simulink model "APCSBussedVersion"  (R2023a)
settings: Solver=VariableStepAuto  StartTime=0.0  StopTime=10.0  RelTol=1e-3
settings Model: Creator=asd19005  LastModifiedBy=asd19005

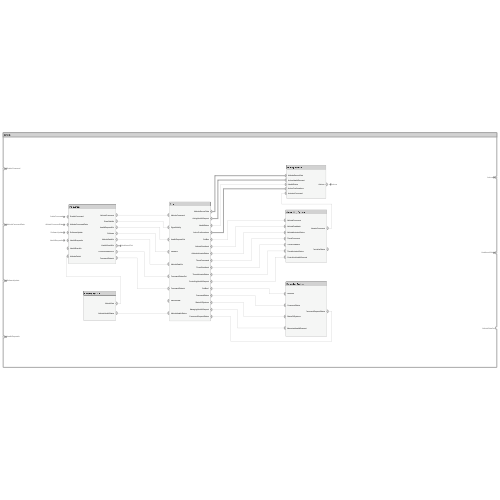
[thumbnail: Simulink's stored preview of the top-level diagram]
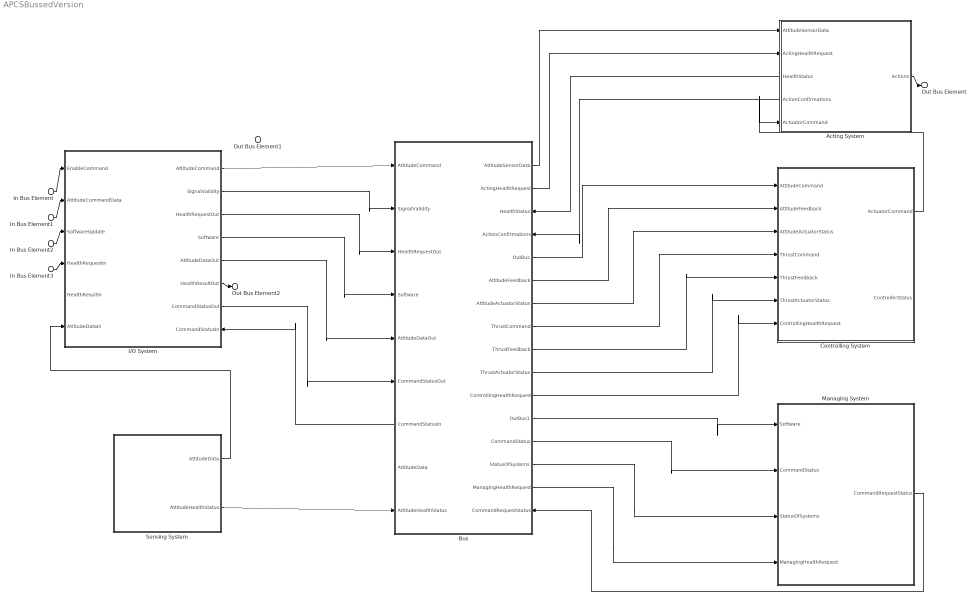
== system APCSBussedVersion ==
  In Bus Element : Inport  PortName=EnableCommand
  In Bus Element1 : Inport  Port=2  PortName=AttitudeCommandData
  In Bus Element2 : Inport  Port=3  PortName=SoftwareUpdate
  In Bus Element3 : Inport  Port=4  PortName=HealthRequestIn
  Acting System : Subsystem
      settings: PortSchema="{\"entries\":[{\"content\":{\"headerSize\":26,\"margin\":15,\"minimumSpacing\":25,\"sides\":[{\"content\":{\"connectorIds\":[\"In1\",\"In2\",\"Out3\",\"Out2\",\"In3\"]},\"type\":\"ConnectorPlacement.EquallySpacedRectSide\",\"uuid\":\"fe9a0813-768f-43cf-a7a7-a35f6718a35e\"},{\"content\":{\"connectorIds\":[\"Out1\"],\"side\":\"RIGHT\"},\"type\":\"ConnectorPlacement.EquallySpacedRectSide\",\"uuid\":\"83a5fda2-f793-4516-8295-8e256804f86f\"},{\"content\":{\"side\":\"TOP\"},\"type\":\"ConnectorPlacement.EquallySpacedRectSide\",\"uuid\":\"9f7bc7bd-a98b-401f-acf1-cfd6a0f445f8\"}]},\"type\":\"ConnectorPlacement.EquallySpacedConnector\",\"uuid\":\"2641b729-a1f9-4d54-83a2-7f405081950a\"}],\"packageUris\":[\"http://schema.mathworks.com/mf0/Connector/R2020b\"],\"version\":\"1.0\"}"
  Bus : Subsystem
      settings: PortSchema="{\"entries\":[{\"content\":{\"headerSize\":26,\"margin\":15,\"minimumSpacing\":25,\"sides\":[{\"content\":{\"connectorIds\":[\"In4\",\"In5\",\"In6\",\"In7\",\"In8\",\"In9\",\"Out1\",\"In10\",\"In11\"]},\"type\":\"ConnectorPlacement.EquallySpacedRectSide\",\"uuid\":\"fe9a0813-768f-43cf-a7a7-a35f6718a35e\"},{\"content\":{\"connectorIds\":[\"Out2\",\"Out3\",\"In2\",\"In3\",\"Out4\",\"Out5\",\"Out6\",\"Out7\",\"Out8\",\"Out9\",\"Out10\",\"Out11\",\"Out12\",\"Out13\",\"Out14\",\"In1\"],\"side\":\"RIGHT\"},\"type\":\"ConnectorPlacement.EquallySpacedRectSide\",\"uuid\":\"83a5fda2-f793-4516-8295-8e256804f86f\"},{\"content\":{\"side\":\"TOP\"},\"type\":\"ConnectorPlacement.EquallySpacedRectSide\",\"uuid\":\"9f7bc7bd-a98b-401f-acf1-cfd6a0f445f8\"},{\"content\":{\"side\":\"BOTTOM\"},\"type\":\"ConnectorPlacement.EquallySpacedRectSide\",\"uuid\":\"63235dc2-7ea6-46cb-9adb-862789535c96\"}]},\"type\":\"ConnectorPlacement.EquallySpacedConnector\",\"uuid\":\"2641b729-a1f9-4d54-83a2-7f405081950a\"}],\"packageUris\":[\"http://schema.mathworks.com/mf0/Connector/R2020b\"],\"version\":\"1.0\"}"
  Controlling System : Subsystem
      settings: PortSchema="{\"entries\":[{\"content\":{\"headerSize\":26,\"margin\":15,\"minimumSpacing\":25,\"sides\":[{\"content\":{\"connectorIds\":[\"In1\",\"In5\",\"In3\",\"In2\",\"In6\",\"In4\",\"In7\"]},\"type\":\"ConnectorPlacement.EquallySpacedRectSide\",\"uuid\":\"fe9a0813-768f-43cf-a7a7-a35f6718a35e\"},{\"content\":{\"connectorIds\":[\"Out1\",\"Out2\"],\"side\":\"RIGHT\"},\"type\":\"ConnectorPlacement.EquallySpacedRectSide\",\"uuid\":\"83a5fda2-f793-4516-8295-8e256804f86f\"},{\"content\":{\"side\":\"TOP\"},\"type\":\"ConnectorPlacement.EquallySpacedRectSide\",\"uuid\":\"9f7bc7bd-a98b-401f-acf1-cfd6a0f445f8\"}]},\"type\":\"ConnectorPlacement.EquallySpacedConnector\",\"uuid\":\"2641b729-a1f9-4d54-83a2-7f405081950a\"}],\"packageUris\":[\"http://schema.mathworks.com/mf0/Connector/R2020b\"],\"version\":\"1.0\"}"
  I/O System : Subsystem
      settings: PortSchema="{\"entries\":[{\"content\":{\"headerSize\":26,\"margin\":15,\"minimumSpacing\":25,\"sides\":[{\"content\":{\"connectorIds\":[\"In1\",\"In2\",\"In3\",\"In4\",\"In5\",\"In6\"]},\"type\":\"ConnectorPlacement.EquallySpacedRectSide\",\"uuid\":\"fe9a0813-768f-43cf-a7a7-a35f6718a35e\"},{\"content\":{\"connectorIds\":[\"Out1\",\"Out2\",\"Out4\",\"Out3\",\"Out5\",\"Out6\",\"Out7\",\"In7\"],\"side\":\"RIGHT\"},\"type\":\"ConnectorPlacement.EquallySpacedRectSide\",\"uuid\":\"83a5fda2-f793-4516-8295-8e256804f86f\"},{\"content\":{\"side\":\"TOP\"},\"type\":\"ConnectorPlacement.EquallySpacedRectSide\",\"uuid\":\"9f7bc7bd-a98b-401f-acf1-cfd6a0f445f8\"}]},\"type\":\"ConnectorPlacement.EquallySpacedConnector\",\"uuid\":\"2641b729-a1f9-4d54-83a2-7f405081950a\"}],\"packageUris\":[\"http://schema.mathworks.com/mf0/Connector/R2020b\"],\"version\":\"1.0\"}"
  Managing System : Subsystem
      settings: PortSchema="{\"entries\":[{\"content\":{\"headerSize\":26,\"margin\":15,\"minimumSpacing\":25,\"sides\":[{\"content\":{\"connectorIds\":[\"In1\",\"In2\",\"In3\",\"In4\"]},\"type\":\"ConnectorPlacement.EquallySpacedRectSide\",\"uuid\":\"fe9a0813-768f-43cf-a7a7-a35f6718a35e\"},{\"content\":{\"connectorIds\":[\"Out1\"],\"side\":\"RIGHT\"},\"type\":\"ConnectorPlacement.EquallySpacedRectSide\",\"uuid\":\"83a5fda2-f793-4516-8295-8e256804f86f\"},{\"content\":{\"side\":\"TOP\"},\"type\":\"ConnectorPlacement.EquallySpacedRectSide\",\"uuid\":\"9f7bc7bd-a98b-401f-acf1-cfd6a0f445f8\"}]},\"type\":\"ConnectorPlacement.EquallySpacedConnector\",\"uuid\":\"2641b729-a1f9-4d54-83a2-7f405081950a\"}],\"packageUris\":[\"http://schema.mathworks.com/mf0/Connector/R2020b\"],\"version\":\"1.0\"}"
  Sensing System : Subsystem
      settings: PortSchema="{\"entries\":[{\"content\":{\"headerSize\":26,\"margin\":15,\"minimumSpacing\":25,\"sides\":[{\"content\":{},\"type\":\"ConnectorPlacement.EquallySpacedRectSide\",\"uuid\":\"fe9a0813-768f-43cf-a7a7-a35f6718a35e\"},{\"content\":{\"connectorIds\":[\"Out1\",\"Out2\"],\"side\":\"RIGHT\"},\"type\":\"ConnectorPlacement.EquallySpacedRectSide\",\"uuid\":\"83a5fda2-f793-4516-8295-8e256804f86f\"},{\"content\":{\"side\":\"TOP\"},\"type\":\"ConnectorPlacement.EquallySpacedRectSide\",\"uuid\":\"9f7bc7bd-a98b-401f-acf1-cfd6a0f445f8\"}]},\"type\":\"ConnectorPlacement.EquallySpacedConnector\",\"uuid\":\"2641b729-a1f9-4d54-83a2-7f405081950a\"}],\"packageUris\":[\"http://schema.mathworks.com/mf0/Connector/R2020b\"],\"version\":\"1.0\"}"
  Out Bus Element : Outport  PortName=Actions
  Out Bus Element2 : Outport  Port=2  PortName=HealthesultOut
  Out Bus Element1 : Outport  Port=3  PortName=AttitudeDataOut
  wires:
  In Bus Element/1 -> I/O System/1(EnableCommand)
  In Bus Element1/1 -> I/O System/2(AttitudeCommandData)
  In Bus Element2/1 -> I/O System/3(SoftwareUpdate)
  In Bus Element3/1 -> I/O System/4(HealthRequestIn)
  Acting System/1(Actions) -> Out Bus Element/1
  I/O System/1(AttitudeCommand) -> Bus/4(AttitudeCommand)
  I/O System/2(SignalValidity) -> Bus/5(SignalValidity)
  I/O System/3(Software) -> Bus/7(Software)
  I/O System/4(HealthRequestOut) -> Bus/6(HealthRequestOut)
  I/O System/5(AttitudeDataOut) -> Bus/8(AttitudeDataOut)
  I/O System/7(CommandStatusOut) -> Bus/9(CommandStatusOut)
  I/O System/6(HealthResultOut) -> Out Bus Element2/1
  Sensing System/2(AttitudeHealthStatus) -> Bus/11(AttitudeHealthStatus)
  Controlling System/1(ActuatorCommand) -> Acting System/3(ActuatorCommand)
  Bus/2(AttitudeSensorData) -> Acting System/1(AttitudeSensorData)
  Sensing System/1(AttitudeData) -> I/O System/6(AttitudeDataIn)
  Bus/3(ActingHealthRequest) -> Acting System/2(ActingHealthRequest)
  Acting System/3(HealthStatus) -> Bus/2(HealthStatus)
  Acting System/2(ActionConfirmations) -> Bus/3(ActionConfirmations)
  Bus/4(OutBus) -> Controlling System/1(AttitudeCommand)
  Bus/5(AttitudeFeedback) -> Controlling System/5(AttitudeFeedback)
  Bus/6(AttitudeActuatorStatus) -> Controlling System/3(AttitudeActuatorStatus)
  Bus/7(ThrustCommand) -> Controlling System/2(ThrustCommand)
  Bus/8(ThrustFeedback) -> Controlling System/6(ThrustFeedback)
  Bus/9(ThrustActuatorStatus) -> Controlling System/4(ThrustActuatorStatus)
  Bus/10(ControllingHealthRequest) -> Controlling System/7(ControllingHealthRequest)
  Bus/12(CommandStatus) -> Managing System/2(CommandStatus)
  Bus/13(StatusOfSystems) -> Managing System/3(StatusOfSystems)
  Bus/14(ManagingHealthRequest) -> Managing System/4(ManagingHealthRequest)
  Bus/11(OutBus1) -> Managing System/1(Software)
  Managing System/1(CommandRequestStatus) -> Bus/1(CommandRequestStatus)
  Bus/1(CommandStatusIn) -> I/O System/7(CommandStatusIn)

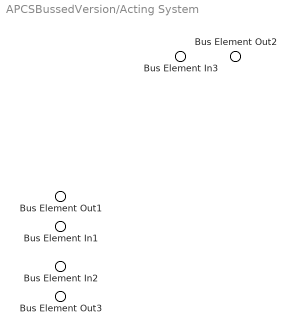
== system APCSBussedVersion/Acting System ==
  Bus Element In1 : Inport  PortName=AttitudeSensorData
  Bus Element In3 : Inport  Port=2  PortName=ActingHealthRequest
  Bus Element In2 : Inport  Port=3  PortName=ActuatorCommand
  Bus Element Out2 : Outport  PortName=Actions
  Bus Element Out1 : Outport  Port=2  PortName=ActionConfirmations
  Bus Element Out3 : Outport  Port=3  PortName=HealthStatus

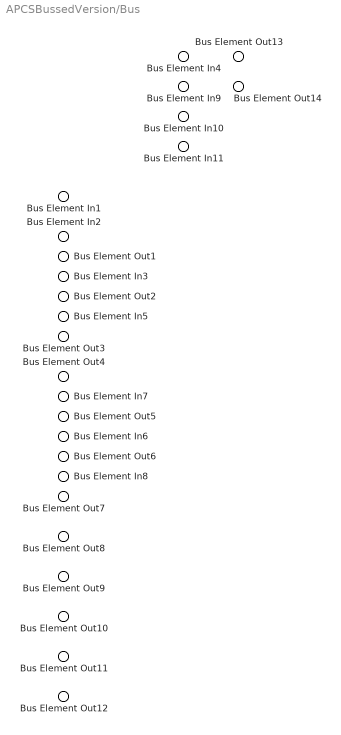
== system APCSBussedVersion/Bus ==
  Bus Element In11 : Inport  PortName=CommandRequestStatus
  Bus Element In9 : Inport  Port=2  PortName=HealthStatus
  Bus Element In10 : Inport  Port=3  PortName=ActionConfirmations
  Bus Element In1 : Inport  Port=4  PortName=AttitudeCommand
  Bus Element In2 : Inport  Port=5  PortName=SignalValidity
  Bus Element In4 : Inport  Port=6  PortName=HealthRequestOut
  Bus Element In3 : Inport  Port=7  PortName=Software
  Bus Element In5 : Inport  Port=8  PortName=AttitudeDataOut
  Bus Element In7 : Inport  Port=9  PortName=CommandStatusOut
  Bus Element In6 : Inport  Port=10  PortName=AttitudeData
  Bus Element In8 : Inport  Port=11  PortName=AttitudeHealthStatus
  Bus Element Out14 : Outport  PortName=CommandStatusIn
  Bus Element Out1 : Outport  Port=2  PortName=AttitudeSensorData
  Bus Element Out2 : Outport  Port=3  PortName=ActingHealthRequest
  Bus Element Out3 : Outport  Port=4  PortName=OutBus
  Bus Element Out4 : Outport  Port=5  PortName=AttitudeFeedback
  Bus Element Out5 : Outport  Port=6  PortName=AttitudeActuatorStatus
  Bus Element Out6 : Outport  Port=7  PortName=ThrustCommand
  Bus Element Out7 : Outport  Port=8  PortName=ThrustFeedback
  Bus Element Out8 : Outport  Port=9  PortName=ThrustActuatorStatus
  Bus Element Out9 : Outport  Port=10  PortName=ControllingHealthRequest
  Bus Element Out13 : Outport  Port=11  PortName=OutBus1
  Bus Element Out10 : Outport  Port=12  PortName=CommandStatus
  Bus Element Out11 : Outport  Port=13  PortName=StatusOfSystems
  Bus Element Out12 : Outport  Port=14  PortName=ManagingHealthRequest

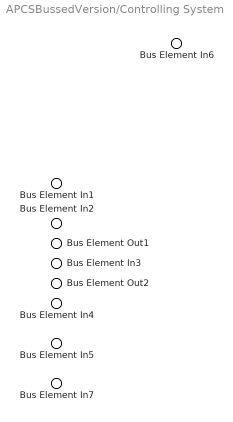
== system APCSBussedVersion/Controlling System ==
  Bus Element In1 : Inport  PortName=AttitudeCommand
  Bus Element In2 : Inport  Port=2  PortName=ThrustCommand
  Bus Element In6 : Inport  Port=3  PortName=AttitudeActuatorStatus
  Bus Element In3 : Inport  Port=4  PortName=ThrustActuatorStatus
  Bus Element In4 : Inport  Port=5  PortName=AttitudeFeedback
  Bus Element In5 : Inport  Port=6  PortName=ThrustFeedback
  Bus Element In7 : Inport  Port=7  PortName=ControllingHealthRequest
  Bus Element Out1 : Outport  PortName=ActuatorCommand
  Bus Element Out2 : Outport  Port=2  PortName=ControllerStatus

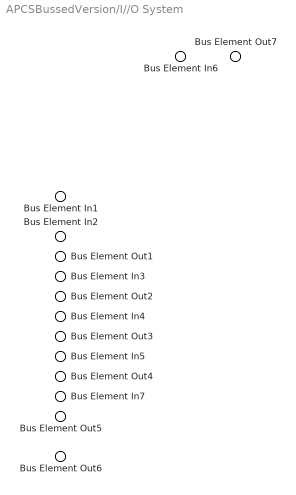
== system APCSBussedVersion/I//O System ==
  Bus Element In1 : Inport  PortName=EnableCommand
  Bus Element In2 : Inport  Port=2  PortName=AttitudeCommandData
  Bus Element In3 : Inport  Port=3  PortName=SoftwareUpdate
  Bus Element In4 : Inport  Port=4  PortName=HealthRequestIn
  Bus Element In6 : Inport  Port=5  PortName=HealthResultIn
  Bus Element In5 : Inport  Port=6  PortName=AttitudeDataIn
  Bus Element In7 : Inport  Port=7  PortName=CommandStatusIn
  Bus Element Out1 : Outport  PortName=AttitudeCommand
  Bus Element Out2 : Outport  Port=2  PortName=SignalValidity
  Bus Element Out3 : Outport  Port=3  PortName=Software
  Bus Element Out4 : Outport  Port=4  PortName=HealthRequestOut
  Bus Element Out5 : Outport  Port=5  PortName=AttitudeDataOut
  Bus Element Out7 : Outport  Port=6  PortName=HealthResultOut
  Bus Element Out6 : Outport  Port=7  PortName=CommandStatusOut

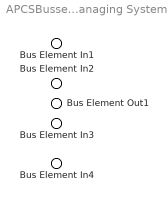
== system APCSBussedVersion/Managing System ==
  Bus Element In1 : Inport  PortName=Software
  Bus Element In2 : Inport  Port=2  PortName=CommandStatus
  Bus Element In3 : Inport  Port=3  PortName=StatusOfSystems
  Bus Element In4 : Inport  Port=4  PortName=ManagingHealthRequest
  Bus Element Out1 : Outport  PortName=CommandRequestStatus

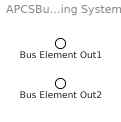
== system APCSBussedVersion/Sensing System ==
  Bus Element Out1 : Outport  PortName=AttitudeData
  Bus Element Out2 : Outport  Port=2  PortName=AttitudeHealthStatus
